simulink model "Test_9_bus_system"  (R2023b)
settings: Solver=VariableStepAuto  StartTime=0.0  StopTime=1  RelTol=1e-3
libraries: spsThreePhaseVIMeasurementLib x15, spsLoadFlowBusLib x9, spsPMUPLLBasedPositiveSequenceLib x6, spsSequenceAnalyzerLib x6, spsThreePhasePISectionLineLib x6, spsThreePhaseFaultLib x6, spsThreePhaseSourceLib x3, spsThreePhaseTransformerTwoWindingsLib x3, spsThreePhaseParallelRLCLoadLib x3, sps_lib x1
settings Model: Creator=korar  LastModifiedBy=korar

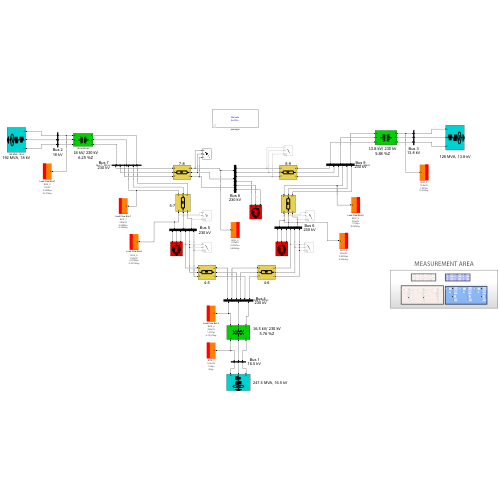
[thumbnail: Simulink's stored preview of the top-level diagram]
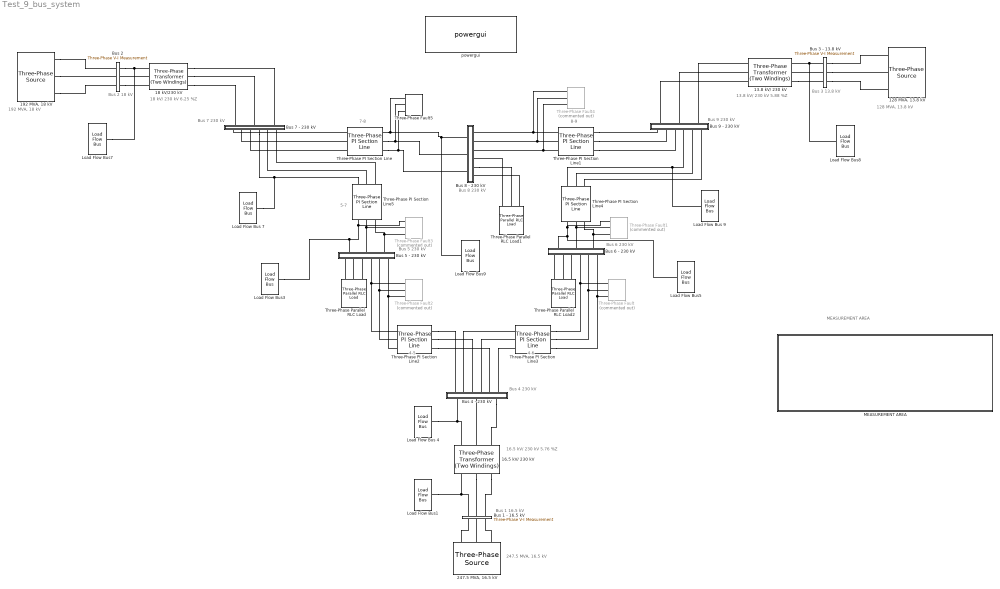
== system Test_9_bus_system ==
  note: MEASUREMENT AREA
  note: Bus 9
      | 230 kV
  note: 5-7
  note: 192 MVA, 18 kV
  note: 128 MVA, 13.8 kV
  note: 247.5 MVA, 16.5 kV
  note: 18 kV/ 230 kV
      | 6.25 %Z
  note: Bus 2
      | 18 kV
  note: Bus 3
      | 13.8 kV
  note: 13.8 kV/ 230 kV
      | 5.88 %Z
  note: Bus 1
      | 16.5 kV
  note: 16.5 kV/ 230 kV
      | 5.76 %Z
  note: 7-8
  note: 8-9
  note: 4-5
  note: 4-6
  note: Bus 7
      | 230 kV
  note: Bus 4
      | 230 kV
  note: Bus 5
      | 230 kV
  note: Bus 6
      | 230 kV
  note: Bus 8
      | 230 kV
  "128 MVA, 13.8 kV" : spsThreePhaseSourceLib/Three-Phase Source  InternalConnection=Yg  VoltagePhases=off  Voltage=(13800)*3.87688  PhaseAngle=72.604  Voltage_phases=[13.8e3 13.8e3 13.8e3]/sqrt(3)  PhaseAngles_phases=[0 -120 +120]  Frequency=50  NonIdealSource=on  SpecifyImpedance=off  Resistance=0.8929  Inductance=16.58e-3  ShortCircuitLevel=100e6  BaseVoltage=13.8e3  XRratio=7  BusType=PQ  Pref=128000000  Qref=11450000  Prefabc=[10e3, 10e3, 10e3]  Qrefabc=[0, 0, 0]  Qmin=-Inf  Qmax=Inf
  13.8 kV/ 230 kV : spsThreePhaseTransformerTwoWindingsLib/Three-Phase Transformer (Two Windings)  Winding1Connection=Yg  Winding2Connection=Yg  CoreType=Three single-phase transformers  SetSaturation=off  Hysteresis=off  DataFile='hysteresis'  SetInitialFlux=off  Measurements=None  UNITS=pu  NominalPower=[ 100e6 , 50 ]  Winding1=[ 13.8e3 , 1e-6 , 0 ]  Winding2=[ 230e3 , 1e-6 , 0.0586 ]  Rm=500  Lm=500  L0=0.5  Saturation=[ 0,0 ; 0.0024,1.2 ; 1.0,1.52 ]  InitialFluxes=[ 0.8 , -0.8 , 0.7 ]  BreakLoop=off  DiscreteSolver=Trapezoidal iterative  DataType=off  TransfoNumber=1
  16.5 kV/ 230 kV : spsThreePhaseTransformerTwoWindingsLib/Three-Phase Transformer (Two Windings)  Winding1Connection=Yg  Winding2Connection=Yg  CoreType=Three single-phase transformers  SetSaturation=off  Hysteresis=off  DataFile='hysteresis'  SetInitialFlux=off  Measurements=None  UNITS=pu  NominalPower=[ 100e6 , 50 ]  Winding1=[ 16.5e3 , 1e-6 , 0 ]  Winding2=[ 230e3 , 1e-6 , 0.0576 ]  Rm=500  Lm=500  L0=0.5  Saturation=[ 0,0 ; 0.0024,1.2 ; 1.0,1.52 ]  InitialFluxes=[ 0.8 , -0.8 , 0.7 ]  BreakLoop=off  DiscreteSolver=Trapezoidal iterative  DataType=off  TransfoNumber=1
  18 kV/230 kV : spsThreePhaseTransformerTwoWindingsLib/Three-Phase Transformer (Two Windings)  Winding1Connection=Yg  Winding2Connection=Yg  CoreType=Three single-phase transformers  SetSaturation=off  Hysteresis=off  DataFile='hysteresis'  SetInitialFlux=off  Measurements=None  UNITS=pu  NominalPower=[ 100e6 , 50 ]  Winding1=[ 18e3 , 1e-6 , 0 ]  Winding2=[ 230e3 , 1e-6 , 0.0625 ]  Rm=500  Lm=500  L0=0.5  Saturation=[ 0,0 ; 0.0024,1.2 ; 1.0,1.52 ]  InitialFluxes=[ 0.8 , -0.8 , 0.7 ]  BreakLoop=off  DiscreteSolver=Trapezoidal iterative  DataType=off  TransfoNumber=1
  "192 MVA, 18 kV" : spsThreePhaseSourceLib/Three-Phase Source  Description=|  InternalConnection=Yg  VoltagePhases=off  Voltage=(18000)*3.48427  PhaseAngle=78.8297  Voltage_phases=[13.8e3 13.8e3 13.8e3]/sqrt(3)  PhaseAngles_phases=[0 -120 +120]  Frequency=50  NonIdealSource=on  SpecifyImpedance=off  Resistance=0.8929  Inductance=16.58e-3  ShortCircuitLevel=100e6  BaseVoltage=18e3  XRratio=7  BusType=PQ  Pref=192000000  Qref=4900000  Prefabc=[10e3, 10e3, 10e3]  Qrefabc=[0, 0, 0]  Qmin=-Inf  Qmax=Inf
      | 60 MVA
      | 13.8 kV
  "247.5 MVA, 16.5 kV" : spsThreePhaseSourceLib/Three-Phase Source  Description=|  InternalConnection=Yg  VoltagePhases=off  Voltage=(16500)*2.16741  PhaseAngle=-2.7069  Voltage_phases=[13.8e3 13.8e3 13.8e3]/sqrt(3)  PhaseAngles_phases=[0 -120 +120]  Frequency=50  NonIdealSource=on  SpecifyImpedance=off  Resistance=0.8929  Inductance=16.58e-3  ShortCircuitLevel=100e6  BaseVoltage=16.5e3  XRratio=7  BusType=swing  Pref=247500000  Qref=27910000  Prefabc=[10e3, 10e3, 10e3]  Qrefabc=[0, 0, 0]  Qmin=-Inf  Qmax=Inf
      | 60 MVA
      | 13.8 kV
  Bus 1 - 16.5 kV : spsThreePhaseVIMeasurementLib/Three-Phase V-I Measurement  VoltageMeasurement=phase-to-ground  SetLabelV=on  LabelV=Vabc_1  Vpu=on  VpuLL=off  CurrentMeasurement=yes  SetLabelI=on  LabelI=Iabc_1  Ipu=on  Pbase=100e6  Vbase=16.5e3  OutputType=Complex  PhasorSimulation=off  PSBequivalent=0
  Bus 2 : spsThreePhaseVIMeasurementLib/Three-Phase V-I Measurement  VoltageMeasurement=phase-to-ground  SetLabelV=on  LabelV=Vabc_2  Vpu=on  VpuLL=off  CurrentMeasurement=yes  SetLabelI=on  LabelI=Iabc_2  Ipu=on  Pbase=100e6  Vbase=18e3  OutputType=Complex  PhasorSimulation=off  PSBequivalent=0
  Bus 3 - 13.8 kV : spsThreePhaseVIMeasurementLib/Three-Phase V-I Measurement  VoltageMeasurement=phase-to-ground  SetLabelV=on  LabelV=Vabc_3  Vpu=on  VpuLL=off  CurrentMeasurement=yes  SetLabelI=on  LabelI=Iabc_3  Ipu=on  Pbase=100e6  Vbase=13.8e3  OutputType=Complex  PhasorSimulation=off  PSBequivalent=0
  Bus 4 - 230 kV : Subsystem
  Bus 5 - 230 kV : Subsystem
  Bus 6 - 230 kV : Subsystem
  Bus 7 - 230 kV : Subsystem
  Bus 8 - 230 kV : Subsystem
  Bus 9 - 230 kV : Subsystem
  Load Flow Bus 4 : spsLoadFlowBusLib/Load Flow Bus  LConnTagsString=a  Phases=single  Connectors=on one side  ID=BUS_4  Vbase=230e3  Vref=1  Vangle=0  VLF=1.007  VLFb=1  VLFc=1  angleLF=-0.1437  angleLFb=0  angleLFc=0
  Load Flow Bus 7 : spsLoadFlowBusLib/Load Flow Bus  LConnTagsString=a  Phases=single  Connectors=on one side  ID=BUS_7  Vbase=230e3  Vref=1  Vangle=0  VLF=0.9982  VLFb=1  VLFc=1  angleLF=9.326  angleLFb=0  angleLFc=0
  Load Flow Bus 9 : spsLoadFlowBusLib/Load Flow Bus  LConnTagsString=a  Phases=single  Connectors=on one side  ID=BUS_9  Vbase=230e3  Vref=1  Vangle=0  VLF=1.019  VLFb=1  VLFc=1  angleLF=8.097  angleLFb=0  angleLFc=0
  Load Flow Bus1 : spsLoadFlowBusLib/Load Flow Bus  LConnTagsString=a  Phases=single  Connectors=on one side  ID=BUS_1  Vbase=16.5e3  Vref=1.04  Vangle=0  VLF=1.04  VLFb=1  VLFc=1  angleLF=0  angleLFb=0  angleLFc=0
  Load Flow Bus3 : spsLoadFlowBusLib/Load Flow Bus  LConnTagsString=a  Phases=single  Connectors=on one side  ID=BUS_5  Vbase=230e3  Vref=1  Vangle=0  VLF=0.9705  VLFb=1  VLFc=1  angleLF=-0.2218  angleLFb=0  angleLFc=0
  Load Flow Bus5 : spsLoadFlowBusLib/Load Flow Bus  LConnTagsString=a  Phases=single  Connectors=on one side  ID=BUS_6  Vbase=230e3  Vref=1  Vangle=0  VLF=0.9908  VLFb=1  VLFc=1  angleLF=0.264  angleLFb=0  angleLFc=0
  Load Flow Bus7 : spsLoadFlowBusLib/Load Flow Bus  LConnTagsString=a  Phases=single  Connectors=on one side  ID=BUS_2  Vbase=18e3  Vref=1.025  Vangle=0  VLF=0.9938  VLFb=1  VLFc=1  angleLF=16.27  angleLFb=0  angleLFc=0
  Load Flow Bus8 : spsLoadFlowBusLib/Load Flow Bus  LConnTagsString=a  Phases=single  Connectors=on one side  ID=BUS_3  Vbase=13.8e3  Vref=1.025  Vangle=0  VLF=1.023  VLFb=1  VLFc=1  angleLF=12.22  angleLFb=0  angleLFc=0
  Load Flow Bus9 : spsLoadFlowBusLib/Load Flow Bus  LConnTagsString=a  Phases=single  Connectors=on one side  ID=BUS_8  Vbase=230e3  Vref=1  Vangle=0  VLF=0.9941  VLFb=1  VLFc=1  angleLF=6.865  angleLFb=0  angleLFc=0
  MEASUREMENT AREA : Subsystem
  Three-Phase PI Section Line : spsThreePhasePISectionLineLib/Three-Phase PI Section Line  LConnTagsString=a|b|c  RConnTagsString=A|B|C  Length=100  Frequency=50  Resistances=[ 0.044965 0.11241]  Inductances="[ 1.01e-3  2.02e-3]"  Capacitances=[7.471e-9 4.394e-9]
  Three-Phase PI Section Line1 : spsThreePhasePISectionLineLib/Three-Phase PI Section Line  LConnTagsString=a|b|c  RConnTagsString=A|B|C  Length=100  Frequency=50  Resistances=[ 0.062951 0.15737]  Inductances="[ 1.414e-3  3.53e-3]"  Capacitances=[10.47e-9 6.15e-9]
  Three-Phase PI Section Line2 : spsThreePhasePISectionLineLib/Three-Phase PI Section Line  LConnTagsString=a|b|c  RConnTagsString=A|B|C  Length=100  Frequency=50  Resistances=[ 0.0529 0.13225]  Inductances="[ 1.192e-3  2.38e-3]"  Capacitances=[8.82e-9 5.188e-9]
  Three-Phase PI Section Line3 : spsThreePhasePISectionLineLib/Three-Phase PI Section Line  LConnTagsString=a|b|c  RConnTagsString=A|B|C  Length=100  Frequency=50  Resistances=[ 0.08993 0.224825]  Inductances="[ 1.29e-3  3.22e-3]"  Capacitances=[7.922e-9 4.74e-9]
  Three-Phase PI Section Line4 : spsThreePhasePISectionLineLib/Three-Phase PI Section Line  LConnTagsString=a|b|c  RConnTagsString=A|B|C  Length=100  Frequency=50  Resistances=[ 0.20631 0.5157]  Inductances="[ 2.38e-3  6.09e-3]"  Capacitances=[17.95e-9 10.55e-9]
  Three-Phase PI Section Line5 : spsThreePhasePISectionLineLib/Three-Phase PI Section Line  LConnTagsString=a|b|c  RConnTagsString=A|B|C  Length=100  Frequency=50  Resistances=[ 0.16928 0.4232]  Inductances="[ 2.259e-3  5.64e-3]"  Capacitances=[15.34e-9 9.025e-9]
  Three-Phase Parallel RLC Load : spsThreePhaseParallelRLCLoadLib/Three-Phase Parallel RLC Load  LConnTagsString=A|B|C  Configuration=Y (grounded)  NominalVoltage=(230000)*0.970466  Vabc=[1e3 1e3 1e3]  Vabcp=[1e3 1e3 1e3]  NominalFrequency=50  UnbalancedPower=off  ActivePower=125000000  InductivePower=50000000  CapacitivePower=0  Pabc=[10e3 9e3 11e3]  QLabc=[100 90 110]  QCabc=[100 90 110]  Pabcp=[10e3 9e3 11e3]  QLabcp=[100 90 110]  QCabcp=[100 90 110]  Measurements=None  LoadType=constant PQ
  Three-Phase Parallel RLC Load1 : spsThreePhaseParallelRLCLoadLib/Three-Phase Parallel RLC Load  LConnTagsString=A|B|C  Configuration=Y (grounded)  NominalVoltage=(230000)*0.994116  Vabc=[1e3 1e3 1e3]  Vabcp=[1e3 1e3 1e3]  NominalFrequency=50  UnbalancedPower=off  ActivePower=100000000  InductivePower=35000000  CapacitivePower=0  Pabc=[10e3 9e3 11e3]  QLabc=[100 90 110]  QCabc=[100 90 110]  Pabcp=[10e3 9e3 11e3]  QLabcp=[100 90 110]  QCabcp=[100 90 110]  Measurements=None  LoadType=constant PQ
  Three-Phase Parallel RLC Load2 : spsThreePhaseParallelRLCLoadLib/Three-Phase Parallel RLC Load  LConnTagsString=A|B|C  Configuration=Y (grounded)  NominalVoltage=(230000)*0.990813  Vabc=[1e3 1e3 1e3]  Vabcp=[1e3 1e3 1e3]  NominalFrequency=50  UnbalancedPower=off  ActivePower=90000000  InductivePower=30000000  CapacitivePower=0  Pabc=[10e3 9e3 11e3]  QLabc=[100 90 110]  QCabc=[100 90 110]  Pabcp=[10e3 9e3 11e3]  QLabcp=[100 90 110]  QCabcp=[100 90 110]  Measurements=None  LoadType=constant PQ
  Three-Phase Fault : spsThreePhaseFaultLib/Three-Phase Fault  Commented=on  InitialStates=0  FaultA=on  FaultB=on  FaultC=on  GroundFault=on  SwitchTimes="[0.6  1]"  External=off  SwitchStatus=NaN  FaultResistance=0.001  GroundResistance=0.01  SnubberResistance=1e6  SnubberCapacitance=inf  Measurements=Fault currents
  Three-Phase Fault1 : spsThreePhaseFaultLib/Three-Phase Fault  Commented=on  InitialStates=0  FaultA=on  FaultB=off  FaultC=off  GroundFault=on  SwitchTimes="[0.6  1]"  External=off  SwitchStatus=NaN  FaultResistance=0.001  GroundResistance=0.01  SnubberResistance=1e6  SnubberCapacitance=inf  Measurements=Fault currents
  Three-Phase Fault2 : spsThreePhaseFaultLib/Three-Phase Fault  Commented=on  InitialStates=0  FaultA=off  FaultB=on  FaultC=on  GroundFault=off  SwitchTimes="[8  10]"  External=off  SwitchStatus=NaN  FaultResistance=0.001  GroundResistance=0.01  SnubberResistance=1e6  SnubberCapacitance=inf  Measurements=Fault currents
  Three-Phase Fault3 : spsThreePhaseFaultLib/Three-Phase Fault  Commented=on  InitialStates=0  FaultA=off  FaultB=on  FaultC=on  GroundFault=off  SwitchTimes="[6/10  1]"  External=off  SwitchStatus=NaN  FaultResistance=0.001  GroundResistance=0.01  SnubberResistance=1e6  SnubberCapacitance=inf  Measurements=Fault currents
  Three-Phase Fault4 : spsThreePhaseFaultLib/Three-Phase Fault  Commented=on  InitialStates=0  FaultA=on  FaultB=on  FaultC=on  GroundFault=off  SwitchTimes="[8  10]"  External=off  SwitchStatus=NaN  FaultResistance=0.001  GroundResistance=0.01  SnubberResistance=1e6  SnubberCapacitance=inf  Measurements=Fault currents
  Three-Phase Fault5 : spsThreePhaseFaultLib/Three-Phase Fault  InitialStates=0  FaultA=off  FaultB=on  FaultC=on  GroundFault=off  SwitchTimes="[0.6  1]"  External=off  SwitchStatus=NaN  FaultResistance=0.001  GroundResistance=0.01  SnubberResistance=1e6  SnubberCapacitance=inf  Measurements=Fault currents
  powergui : sps_lib/powergui  Priority=1  SimulationMode=Discrete  SampleTime=50e-6  frequency=50  Iterations=50  frequencyindice=50  Pbase=100e6  ErrMax=1e-4  UnitsV=kV  UnitsW=MW  buscounter=0  FunctionMessages=off  echomessages=off  EnableUseOfTLC=off  CurrentSourceSwitches=off  DisableSnubberDevices=off  DisableRonSwitches=off  DisableVfSwitches=off  DisplayEquations=off  AutomaticDiscreteSolvers=off  SolverType=Tustin/Backward Euler (TBE)  Interpol=off  ExternalGateDelay=off  methode=off  Ts=100  x0status=blocks  SPID=on  SwTol=0  HookPort=off  NonlinearTolerance=1e-4  nMaxIteration=100  ContinueOnMaxIteration=off  RestoreLinks=warning  ResistiveCurrentMeasurement=off  Frange=[0:2:500]  Ylog=off  Xlog=on  ShowGrid=off  save=off  variable=ZData  structure=0  ZoomFFT=off  StartTime=0.0  cycles=1  DisplayStyle=1  fundamental=60  FreqAxis=off  MaxFrequency=1000  frequencyindicesteady=1  RmsSteady=1  display=off
  connections:
  Bus 3 - 13.8 kV/RConn1 -- "128 MVA, 13.8 kV"/RConn1
  Bus 3 - 13.8 kV/RConn2 -- "128 MVA, 13.8 kV"/RConn2
  Bus 3 - 13.8 kV/RConn3 -- "128 MVA, 13.8 kV"/RConn3
  "247.5 MVA, 16.5 kV"/RConn1 -- Bus 1 - 16.5 kV/RConn1
  "247.5 MVA, 16.5 kV"/RConn2 -- Bus 1 - 16.5 kV/RConn2
  "247.5 MVA, 16.5 kV"/RConn3 -- Bus 1 - 16.5 kV/RConn3
  Three-Phase PI Section Line/LConn1 -- Bus 7 - 230 kV/RConn1
  Three-Phase PI Section Line/LConn2 -- Bus 7 - 230 kV/RConn2
  Three-Phase PI Section Line/LConn3 -- Bus 7 - 230 kV/RConn3
  Bus 7 - 230 kV/RConn4 -- Load Flow Bus 7/LConn1 -- Three-Phase PI Section Line5/LConn1
  Three-Phase PI Section Line5/LConn2 -- Bus 7 - 230 kV/RConn5
  Three-Phase PI Section Line5/LConn3 -- Bus 7 - 230 kV/RConn6
  "192 MVA, 18 kV"/RConn1 -- Bus 2/LConn1
  "192 MVA, 18 kV"/RConn2 -- Bus 2/LConn2
  "192 MVA, 18 kV"/RConn3 -- Bus 2/LConn3
  Three-Phase PI Section Line1/RConn1 -- Bus 9 - 230 kV/LConn1
  Three-Phase PI Section Line1/RConn2 -- Bus 9 - 230 kV/LConn2
  Three-Phase PI Section Line1/RConn3 -- Bus 9 - 230 kV/LConn3
  Three-Phase PI Section Line4/LConn1 -- Load Flow Bus 9/LConn1 -- Bus 9 - 230 kV/LConn4
  Three-Phase PI Section Line4/LConn2 -- Bus 9 - 230 kV/LConn5
  Three-Phase PI Section Line4/LConn3 -- Bus 9 - 230 kV/LConn6
  Three-Phase PI Section Line2/RConn1 -- Bus 4 - 230 kV/RConn1
  Three-Phase PI Section Line3/LConn1 -- Bus 4 - 230 kV/RConn2
  Three-Phase PI Section Line2/RConn2 -- Bus 4 - 230 kV/RConn3
  Three-Phase PI Section Line3/LConn2 -- Bus 4 - 230 kV/RConn4
  Three-Phase PI Section Line2/RConn3 -- Bus 4 - 230 kV/RConn5
  Three-Phase PI Section Line3/LConn3 -- Bus 4 - 230 kV/RConn6
  Three-Phase PI Section Line5/RConn2 -- Bus 5 - 230 kV/LConn2 -- Three-Phase Fault3/LConn2
  Three-Phase PI Section Line2/LConn1 -- Three-Phase Fault2/LConn1 -- Bus 5 - 230 kV/RConn4
  Three-Phase PI Section Line2/LConn2 -- Three-Phase Fault2/LConn2 -- Bus 5 - 230 kV/RConn5
  Three-Phase PI Section Line2/LConn3 -- Three-Phase Fault2/LConn3 -- Bus 5 - 230 kV/RConn6
  Three-Phase PI Section Line4/RConn1 -- Load Flow Bus5/LConn1 -- Bus 6 - 230 kV/LConn1 -- Three-Phase Fault1/LConn1
  Three-Phase PI Section Line4/RConn2 -- Bus 6 - 230 kV/LConn2 -- Three-Phase Fault1/LConn2
  Three-Phase PI Section Line4/RConn3 -- Bus 6 - 230 kV/LConn3 -- Three-Phase Fault1/LConn3
  Three-Phase PI Section Line3/RConn1 -- Three-Phase Fault/LConn1 -- Bus 6 - 230 kV/RConn4
  Three-Phase PI Section Line3/RConn2 -- Three-Phase Fault/LConn2 -- Bus 6 - 230 kV/RConn5
  Three-Phase PI Section Line3/RConn3 -- Three-Phase Fault/LConn3 -- Bus 6 - 230 kV/RConn6
  18 kV/230 kV/RConn2 -- Bus 7 - 230 kV/LConn2
  18 kV/230 kV/RConn1 -- Bus 7 - 230 kV/LConn3
  18 kV/230 kV/RConn3 -- Bus 7 - 230 kV/LConn1
  Bus 2/RConn1 -- Load Flow Bus7/LConn1 -- 18 kV/230 kV/LConn1
  Bus 2/RConn3 -- 18 kV/230 kV/LConn3
  18 kV/230 kV/LConn2 -- Bus 2/RConn2
  Bus 9 - 230 kV/RConn1 -- 13.8 kV/ 230 kV/RConn3
  Bus 3 - 13.8 kV/LConn1 -- Load Flow Bus8/LConn1 -- 13.8 kV/ 230 kV/LConn1
  Bus 3 - 13.8 kV/LConn2 -- 13.8 kV/ 230 kV/LConn2
  13.8 kV/ 230 kV/LConn3 -- Bus 3 - 13.8 kV/LConn3
  13.8 kV/ 230 kV/RConn1 -- Bus 9 - 230 kV/RConn3
  13.8 kV/ 230 kV/RConn2 -- Bus 9 - 230 kV/RConn2
  16.5 kV/ 230 kV/RConn2 -- Bus 4 - 230 kV/LConn2
  16.5 kV/ 230 kV/RConn1 -- Load Flow Bus 4/LConn1 -- Bus 4 - 230 kV/LConn1
  Bus 4 - 230 kV/LConn3 -- 16.5 kV/ 230 kV/RConn3
  16.5 kV/ 230 kV/LConn2 -- Bus 1 - 16.5 kV/LConn2
  16.5 kV/ 230 kV/LConn3 -- Bus 1 - 16.5 kV/LConn3
  Bus 1 - 16.5 kV/LConn1 -- Load Flow Bus1/LConn1 -- 16.5 kV/ 230 kV/LConn1
  Three-Phase PI Section Line/RConn1 -- Three-Phase Fault5/LConn1 -- Load Flow Bus9/LConn1 -- Bus 8 - 230 kV/LConn1
  Three-Phase PI Section Line1/LConn1 -- Three-Phase Fault4/LConn1 -- Bus 8 - 230 kV/RConn1
  Three-Phase PI Section Line/RConn2 -- Three-Phase Fault5/LConn2 -- Bus 8 - 230 kV/LConn2
  Three-Phase PI Section Line1/LConn2 -- Three-Phase Fault4/LConn2 -- Bus 8 - 230 kV/RConn2
  Three-Phase PI Section Line/RConn3 -- Three-Phase Fault5/LConn3 -- Bus 8 - 230 kV/LConn3
  Three-Phase PI Section Line1/LConn3 -- Three-Phase Fault4/LConn3 -- Bus 8 - 230 kV/RConn3
  Bus 5 - 230 kV/LConn1 -- Load Flow Bus3/LConn1 -- Three-Phase Fault3/LConn1 -- Three-Phase PI Section Line5/RConn1
  Bus 5 - 230 kV/LConn3 -- Three-Phase PI Section Line5/RConn3 -- Three-Phase Fault3/LConn3
  Three-Phase Parallel RLC Load/LConn1 -- Bus 5 - 230 kV/RConn1
  Three-Phase Parallel RLC Load/LConn2 -- Bus 5 - 230 kV/RConn2
  Three-Phase Parallel RLC Load/LConn3 -- Bus 5 - 230 kV/RConn3
  Three-Phase Parallel RLC Load1/LConn1 -- Bus 8 - 230 kV/RConn4
  Bus 8 - 230 kV/RConn5 -- Three-Phase Parallel RLC Load1/LConn2
  Three-Phase Parallel RLC Load1/LConn3 -- Bus 8 - 230 kV/RConn6
  Three-Phase Parallel RLC Load2/LConn1 -- Bus 6 - 230 kV/RConn1
  Three-Phase Parallel RLC Load2/LConn2 -- Bus 6 - 230 kV/RConn2
  Three-Phase Parallel RLC Load2/LConn3 -- Bus 6 - 230 kV/RConn3

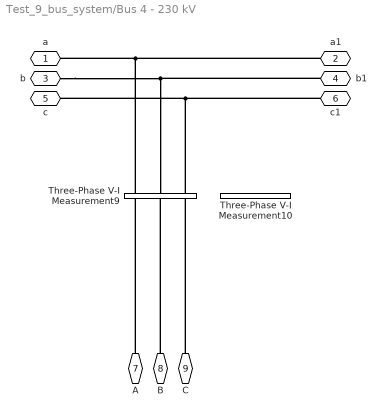
== system Test_9_bus_system/Bus 4 - 230 kV ==
  Three-Phase V-I Measurement10 : spsThreePhaseVIMeasurementLib/Three-Phase V-I Measurement  VoltageMeasurement=phase-to-ground  SetLabelV=on  LabelV=Vabc_42  Vpu=on  VpuLL=off  CurrentMeasurement=yes  SetLabelI=on  LabelI=Iabc_42  Ipu=on  Pbase=100e6  Vbase=230e3  OutputType=Complex  PhasorSimulation=off  PSBequivalent=0
  Three-Phase V-I Measurement9 : spsThreePhaseVIMeasurementLib/Three-Phase V-I Measurement  VoltageMeasurement=phase-to-ground  SetLabelV=on  LabelV=Vabc_41  Vpu=on  VpuLL=off  CurrentMeasurement=yes  SetLabelI=on  LabelI=Iabc_41  Ipu=on  Pbase=100e6  Vbase=230e3  OutputType=Complex  PhasorSimulation=off  PSBequivalent=0
  a : PMIOPort  Side=Right
  a1 : PMIOPort  Port=2  Side=Right
  b : PMIOPort  Port=3  Side=Right
  b1 : PMIOPort  Port=4  Side=Right
  c : PMIOPort  Port=5  Side=Right
  c1 : PMIOPort  Port=6  Side=Right
  A : PMIOPort  Port=7  Side=Left
  B : PMIOPort  Port=8  Side=Left
  C : PMIOPort  Port=9  Side=Left
  connections:
  B/RConn1 -- Three-Phase V-I Measurement9/LConn2
  C/RConn1 -- Three-Phase V-I Measurement9/LConn3
  Three-Phase V-I Measurement9/RConn3 -- c1/RConn1 -- c/RConn1
  A/RConn1 -- Three-Phase V-I Measurement9/LConn1
  b/RConn1 -- b1/RConn1 -- Three-Phase V-I Measurement9/RConn2
  Three-Phase V-I Measurement9/RConn1 -- a1/RConn1 -- a/RConn1

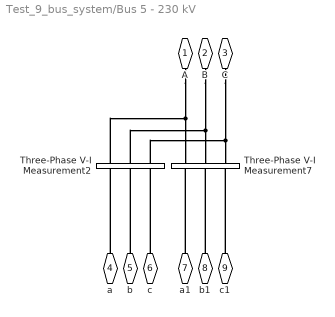
== system Test_9_bus_system/Bus 5 - 230 kV ==
  Three-Phase V-I Measurement2 : spsThreePhaseVIMeasurementLib/Three-Phase V-I Measurement  VoltageMeasurement=phase-to-ground  SetLabelV=on  LabelV=Vabc_51  Vpu=on  VpuLL=off  CurrentMeasurement=yes  SetLabelI=on  LabelI=Iabc_51  Ipu=on  Pbase=100e6  Vbase=230e3  OutputType=Complex  PhasorSimulation=off  PSBequivalent=0
  Three-Phase V-I Measurement7 : spsThreePhaseVIMeasurementLib/Three-Phase V-I Measurement  VoltageMeasurement=phase-to-ground  SetLabelV=on  LabelV=Vabc_52  Vpu=on  VpuLL=off  CurrentMeasurement=yes  SetLabelI=on  LabelI=Iabc_52  Ipu=on  Pbase=100e6  Vbase=230e3  OutputType=Complex  PhasorSimulation=off  PSBequivalent=0
  A : PMIOPort  Side=Left
  B : PMIOPort  Port=2  Side=Left
  C : PMIOPort  Port=3  Side=Left
  a : PMIOPort  Port=4  Side=Right
  b : PMIOPort  Port=5  Side=Right
  c : PMIOPort  Port=6  Side=Right
  a1 : PMIOPort  Port=7  Side=Right
  b1 : PMIOPort  Port=8  Side=Right
  c1 : PMIOPort  Port=9  Side=Right
  connections:
  B/RConn1 -- Three-Phase V-I Measurement2/LConn2 -- Three-Phase V-I Measurement7/LConn2
  b/RConn1 -- Three-Phase V-I Measurement2/RConn2
  A/RConn1 -- Three-Phase V-I Measurement2/LConn1 -- Three-Phase V-I Measurement7/LConn1
  a/RConn1 -- Three-Phase V-I Measurement2/RConn1
  a1/RConn1 -- Three-Phase V-I Measurement7/RConn1
  c1/RConn1 -- Three-Phase V-I Measurement7/RConn3
  C/RConn1 -- Three-Phase V-I Measurement2/LConn3 -- Three-Phase V-I Measurement7/LConn3
  b1/RConn1 -- Three-Phase V-I Measurement7/RConn2
  c/RConn1 -- Three-Phase V-I Measurement2/RConn3

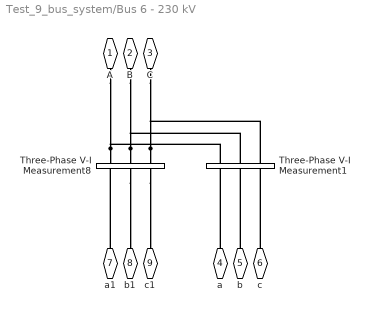
== system Test_9_bus_system/Bus 6 - 230 kV ==
  Three-Phase V-I Measurement1 : spsThreePhaseVIMeasurementLib/Three-Phase V-I Measurement  VoltageMeasurement=phase-to-ground  SetLabelV=on  LabelV=Vabc_62  Vpu=on  VpuLL=off  CurrentMeasurement=yes  SetLabelI=on  LabelI=Iabc_62  Ipu=on  Pbase=100e6  Vbase=230e3  OutputType=Complex  PhasorSimulation=off  PSBequivalent=0
  Three-Phase V-I Measurement8 : spsThreePhaseVIMeasurementLib/Three-Phase V-I Measurement  VoltageMeasurement=phase-to-ground  SetLabelV=on  LabelV=Vabc_61  Vpu=on  VpuLL=off  CurrentMeasurement=yes  SetLabelI=on  LabelI=Iabc_61  Ipu=on  Pbase=100e6  Vbase=230e3  OutputType=Complex  PhasorSimulation=off  PSBequivalent=0
  A : PMIOPort  Side=Left
  B : PMIOPort  Port=2  Side=Left
  C : PMIOPort  Port=3  Side=Left
  a : PMIOPort  Port=4  Side=Right
  b : PMIOPort  Port=5  Side=Right
  c : PMIOPort  Port=6  Side=Right
  a1 : PMIOPort  Port=7  Side=Right
  b1 : PMIOPort  Port=8  Side=Right
  c1 : PMIOPort  Port=9  Side=Right
  connections:
  Three-Phase V-I Measurement8/LConn2 -- B/RConn1 -- Three-Phase V-I Measurement1/LConn2
  Three-Phase V-I Measurement8/LConn1 -- A/RConn1 -- Three-Phase V-I Measurement1/LConn1
  b/RConn1 -- Three-Phase V-I Measurement1/RConn2
  Three-Phase V-I Measurement8/LConn3 -- C/RConn1 -- Three-Phase V-I Measurement1/LConn3
  a/RConn1 -- Three-Phase V-I Measurement1/RConn1
  Three-Phase V-I Measurement8/RConn3 -- c1/RConn1
  Three-Phase V-I Measurement8/RConn2 -- b1/RConn1
  c/RConn1 -- Three-Phase V-I Measurement1/RConn3
  a1/RConn1 -- Three-Phase V-I Measurement8/RConn1

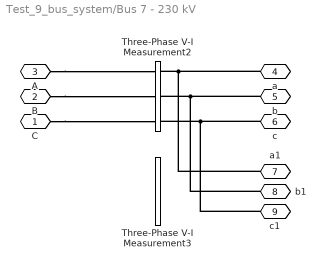
== system Test_9_bus_system/Bus 7 - 230 kV ==
  Three-Phase V-I Measurement2 : spsThreePhaseVIMeasurementLib/Three-Phase V-I Measurement  VoltageMeasurement=phase-to-ground  SetLabelV=on  LabelV=Vabc_71  Vpu=on  VpuLL=off  CurrentMeasurement=yes  SetLabelI=on  LabelI=Iabc_71  Ipu=on  Pbase=100e6  Vbase=230e3  OutputType=Complex  PhasorSimulation=off  PSBequivalent=0
  Three-Phase V-I Measurement3 : spsThreePhaseVIMeasurementLib/Three-Phase V-I Measurement  VoltageMeasurement=phase-to-ground  SetLabelV=on  LabelV=Vabc_72  Vpu=on  VpuLL=off  CurrentMeasurement=yes  SetLabelI=on  LabelI=Iabc_72  Ipu=on  Pbase=100e6  Vbase=230e3  OutputType=Complex  PhasorSimulation=off  PSBequivalent=0
  C : PMIOPort  Side=Left
  B : PMIOPort  Port=2  Side=Left
  A : PMIOPort  Port=3  Side=Left
  a : PMIOPort  Port=4  Side=Right
  b : PMIOPort  Port=5  Side=Right
  c : PMIOPort  Port=6  Side=Right
  a1 : PMIOPort  Port=7  Side=Right
  b1 : PMIOPort  Port=8  Side=Right
  c1 : PMIOPort  Port=9  Side=Right
  connections:
  C/RConn1 -- Three-Phase V-I Measurement2/LConn3
  a/RConn1 -- a1/RConn1 -- Three-Phase V-I Measurement2/RConn1
  A/RConn1 -- Three-Phase V-I Measurement2/LConn1
  b/RConn1 -- b1/RConn1 -- Three-Phase V-I Measurement2/RConn2
  B/RConn1 -- Three-Phase V-I Measurement2/LConn2
  c/RConn1 -- c1/RConn1 -- Three-Phase V-I Measurement2/RConn3

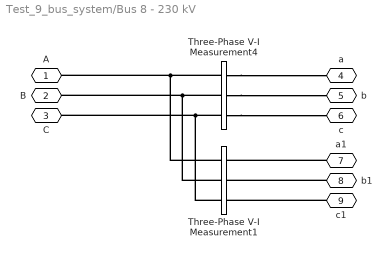
== system Test_9_bus_system/Bus 8 - 230 kV ==
  Three-Phase V-I Measurement1 : spsThreePhaseVIMeasurementLib/Three-Phase V-I Measurement  VoltageMeasurement=phase-to-ground  SetLabelV=on  LabelV=Vabc_82  Vpu=on  VpuLL=off  CurrentMeasurement=yes  SetLabelI=on  LabelI=Iabc_82  Ipu=on  Pbase=100e6  Vbase=230e3  OutputType=Complex  PhasorSimulation=off  PSBequivalent=0
  Three-Phase V-I Measurement4 : spsThreePhaseVIMeasurementLib/Three-Phase V-I Measurement  VoltageMeasurement=phase-to-ground  SetLabelV=on  LabelV=Vabc_81  Vpu=on  VpuLL=off  CurrentMeasurement=yes  SetLabelI=on  LabelI=Iabc_81  Ipu=on  Pbase=100e6  Vbase=230e3  OutputType=Complex  PhasorSimulation=off  PSBequivalent=0
  A : PMIOPort  Side=Left
  B : PMIOPort  Port=2  Side=Left
  C : PMIOPort  Port=3  Side=Left
  a : PMIOPort  Port=4  Side=Right
  b : PMIOPort  Port=5  Side=Right
  c : PMIOPort  Port=6  Side=Right
  a1 : PMIOPort  Port=7  Side=Right
  b1 : PMIOPort  Port=8  Side=Right
  c1 : PMIOPort  Port=9  Side=Right
  connections:
  Three-Phase V-I Measurement4/LConn1 -- A/RConn1 -- Three-Phase V-I Measurement1/LConn1
  Three-Phase V-I Measurement4/RConn1 -- a/RConn1
  Three-Phase V-I Measurement4/LConn3 -- C/RConn1 -- Three-Phase V-I Measurement1/LConn3
  Three-Phase V-I Measurement4/LConn2 -- B/RConn1 -- Three-Phase V-I Measurement1/LConn2
  Three-Phase V-I Measurement4/RConn3 -- c/RConn1
  Three-Phase V-I Measurement4/RConn2 -- b/RConn1
  a1/RConn1 -- Three-Phase V-I Measurement1/RConn1
  b1/RConn1 -- Three-Phase V-I Measurement1/RConn2
  c1/RConn1 -- Three-Phase V-I Measurement1/RConn3

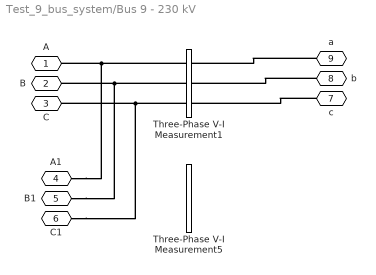
== system Test_9_bus_system/Bus 9 - 230 kV ==
  Three-Phase V-I Measurement1 : spsThreePhaseVIMeasurementLib/Three-Phase V-I Measurement  VoltageMeasurement=phase-to-ground  SetLabelV=on  LabelV=Vabc_91  Vpu=on  VpuLL=off  CurrentMeasurement=yes  SetLabelI=on  LabelI=Iabc_91  Ipu=on  Pbase=100e6  Vbase=230e3  OutputType=Complex  PhasorSimulation=off  PSBequivalent=0
  Three-Phase V-I Measurement5 : spsThreePhaseVIMeasurementLib/Three-Phase V-I Measurement  VoltageMeasurement=phase-to-ground  SetLabelV=on  LabelV=Vabc_92  Vpu=on  VpuLL=off  CurrentMeasurement=yes  SetLabelI=on  LabelI=Iabc_92  Ipu=on  Pbase=100e6  Vbase=230e3  OutputType=Complex  PhasorSimulation=off  PSBequivalent=0
  A : PMIOPort  Side=Left
  B : PMIOPort  Port=2  Side=Left
  C : PMIOPort  Port=3  Side=Left
  A1 : PMIOPort  Port=4  Side=Left
  B1 : PMIOPort  Port=5  Side=Left
  C1 : PMIOPort  Port=6  Side=Left
  c : PMIOPort  Port=7  Side=Right
  b : PMIOPort  Port=8  Side=Right
  a : PMIOPort  Port=9  Side=Right
  connections:
  Three-Phase V-I Measurement1/LConn1 -- A1/RConn1 -- A/RConn1
  b/RConn1 -- Three-Phase V-I Measurement1/RConn2
  Three-Phase V-I Measurement1/LConn3 -- C1/RConn1 -- C/RConn1
  c/RConn1 -- Three-Phase V-I Measurement1/RConn3
  a/RConn1 -- Three-Phase V-I Measurement1/RConn1
  Three-Phase V-I Measurement1/LConn2 -- B1/RConn1 -- B/RConn1

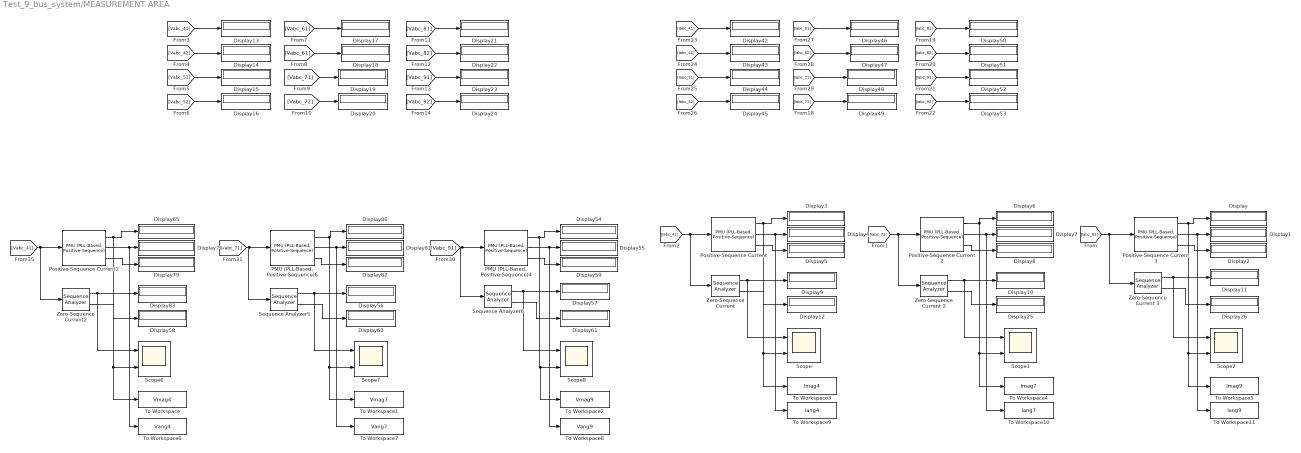
== system Test_9_bus_system/MEASUREMENT AREA ==
  Display{,1..26,42..61,65,76,79..83} (54 alike) : Display
  "PMU (PLL-Based, Positive-Sequence)4" : spsPMUPLLBasedPositiveSequenceLib/PMU (PLL-Based, Positive-Sequence)  nominalFrequency=50  samplingRate=64  reportingFactor=1
      settings: LibrarySourceBlock=|
      | sps_lib/Sensors and Measurements/PMU
      | (PLL-Based,
      | Positive-Sequence)
  "PMU (PLL-Based, Positive-Sequence)6" : spsPMUPLLBasedPositiveSequenceLib/PMU (PLL-Based, Positive-Sequence)  nominalFrequency=50  samplingRate=64  reportingFactor=1
      settings: LibrarySourceBlock=|
      | sps_lib/Sensors and Measurements/PMU
      | (PLL-Based,
      | Positive-Sequence)
  Positive-Sequence Current : spsPMUPLLBasedPositiveSequenceLib/PMU (PLL-Based, Positive-Sequence)  nominalFrequency=50  samplingRate=64  reportingFactor=1
      settings: LibrarySourceBlock=|
      | sps_lib/Sensors and Measurements/PMU
      | (PLL-Based,
      | Positive-Sequence)
  Positive-Sequence Current 2 : spsPMUPLLBasedPositiveSequenceLib/PMU (PLL-Based, Positive-Sequence)  nominalFrequency=50  samplingRate=64  reportingFactor=1
      settings: LibrarySourceBlock=|
      | sps_lib/Sensors and Measurements/PMU
      | (PLL-Based,
      | Positive-Sequence)
  Positive-Sequence Current 3 : spsPMUPLLBasedPositiveSequenceLib/PMU (PLL-Based, Positive-Sequence)  nominalFrequency=50  samplingRate=64  reportingFactor=1
      settings: LibrarySourceBlock=|
      | sps_lib/Sensors and Measurements/PMU
      | (PLL-Based,
      | Positive-Sequence)
  Positive-Sequence Current2 : spsPMUPLLBasedPositiveSequenceLib/PMU (PLL-Based, Positive-Sequence)  nominalFrequency=50  samplingRate=64  reportingFactor=1
      settings: LibrarySourceBlock=|
      | sps_lib/Sensors and Measurements/PMU
      | (PLL-Based,
      | Positive-Sequence)
  Scope{,1..2,6..8} (6 alike) : Scope  NumInputPorts=2
  Sequence Analyzer5 : spsSequenceAnalyzerLib/Sequence Analyzer  Freq=50  n=1  seq=Zero  InInit=[1, 0]  Ts=0
      settings: LibrarySourceBlock=sps_lib/Sensors and Measurements/Sequence Analyzer
  Sequence Analyzer6 : spsSequenceAnalyzerLib/Sequence Analyzer  Freq=50  n=1  seq=Zero  InInit=[1, 0]  Ts=0
      settings: LibrarySourceBlock=sps_lib/Sensors and Measurements/Sequence Analyzer
  To Workspace : ToWorkspace  VariableName=Vmag4  SaveFormat=Timeseries  SampleTime=0.1
      settings: Decimation=3
  To Workspace1 : ToWorkspace  VariableName=Vmag7  SaveFormat=Timeseries  SampleTime=0.1
      settings: Decimation=3
  To Workspace10 : ToWorkspace  VariableName=Iang7  SaveFormat=Timeseries  SampleTime=0.1
      settings: Decimation=3
  To Workspace11 : ToWorkspace  VariableName=Iang9  SaveFormat=Timeseries  SampleTime=0.1
      settings: Decimation=3
  To Workspace2 : ToWorkspace  VariableName=Vmag9  SaveFormat=Timeseries  SampleTime=0.1
      settings: Decimation=3
  To Workspace3 : ToWorkspace  VariableName=Imag4  SaveFormat=Timeseries  SampleTime=0.1
      settings: Decimation=3
  To Workspace4 : ToWorkspace  VariableName=Imag7  SaveFormat=Timeseries  SampleTime=0.1
      settings: Decimation=3
  To Workspace5 : ToWorkspace  VariableName=Imag9  SaveFormat=Timeseries  SampleTime=0.1
      settings: Decimation=3
  To Workspace6 : ToWorkspace  VariableName=Vang4  SaveFormat=Timeseries  SampleTime=0.1
      settings: Decimation=3
  To Workspace7 : ToWorkspace  VariableName=Vang7  SaveFormat=Timeseries  SampleTime=0.1
      settings: Decimation=3
  To Workspace8 : ToWorkspace  VariableName=Vang9  SaveFormat=Timeseries  SampleTime=0.1
      settings: Decimation=3
  To Workspace9 : ToWorkspace  VariableName=Iang4  SaveFormat=Timeseries  SampleTime=0.1
      settings: Decimation=3
  Zero-Sequence Current : spsSequenceAnalyzerLib/Sequence Analyzer  Freq=50  n=1  seq=Zero  InInit=[1, 0]  Ts=0
      settings: LibrarySourceBlock=sps_lib/Sensors and Measurements/Sequence Analyzer
  Zero-Sequence Current 2 : spsSequenceAnalyzerLib/Sequence Analyzer  Freq=50  n=1  seq=Zero  InInit=[1, 0]  Ts=0
      settings: LibrarySourceBlock=sps_lib/Sensors and Measurements/Sequence Analyzer
  Zero-Sequence Current 3 : spsSequenceAnalyzerLib/Sequence Analyzer  Freq=50  n=1  seq=Zero  InInit=[1, 0]  Ts=0
      settings: LibrarySourceBlock=sps_lib/Sensors and Measurements/Sequence Analyzer
  Zero-Sequence Current2 : spsSequenceAnalyzerLib/Sequence Analyzer  Freq=50  n=1  seq=Zero  InInit=[1, 0]  Ts=0
      settings: LibrarySourceBlock=sps_lib/Sensors and Measurements/Sequence Analyzer
  wires:
  Positive-Sequence Current 3/3 -> Display2/1
  [Vabc_71] -> Display19/1
  [Iabc_71] -> Zero-Sequence Current 2/1, Positive-Sequence Current 2/1
  Positive-Sequence Current 3/2 -> To Workspace11/1, Display1/1
  [Vabc_81] -> Display21/1
  Positive-Sequence Current/1 -> To Workspace3/1, Scope/2, Display3/1
  Positive-Sequence Current 2/2 -> To Workspace10/1, Display7/1
  Positive-Sequence Current/2 -> To Workspace9/1, Display4/1
  [Vabc_42] -> Display14/1
  [Vabc_51] -> Display15/1
  [Iabc_41] -> Zero-Sequence Current/1, Positive-Sequence Current/1
  [Vabc_91] -> Display23/1
  Zero-Sequence Current 2/2 -> Display25/1
  Positive-Sequence Current 2/3 -> Display8/1
  [Iabc_91] -> Zero-Sequence Current 3/1, Positive-Sequence Current 3/1
  [Vabc_61] -> Display17/1
  Zero-Sequence Current/1 -> Scope/1, Display9/1
  [Vabc_41] -> Display13/1
  [Vabc_72] -> Display20/1
  [Vabc_92] -> Display24/1
  [Vabc_52] -> Display16/1
  Positive-Sequence Current/3 -> Display5/1
  [Vabc_82] -> Display22/1
  [Vabc_61] -> Display18/1
  Zero-Sequence Current/2 -> Display12/1
  Zero-Sequence Current 3/2 -> Display26/1
  Positive-Sequence Current 2/1 -> To Workspace4/1, Scope1/2, Display6/1
  Zero-Sequence Current 2/1 -> Scope1/1, Display10/1
  Positive-Sequence Current 3/1 -> To Workspace5/1, Scope2/2, Display/1
  Zero-Sequence Current 3/1 -> Scope2/1, Display11/1
  [Iabc_91] -> Display52/1
  [Iabc_82] -> Display51/1
  [Iabc_41] -> Display43/1
  [Iabc_51] -> Display44/1
  [Iabc_61] -> Display46/1
  [Iabc_81] -> Display50/1
  [Iabc_52] -> Display45/1
  [Iabc_62] -> Display47/1
  [Iabc_71] -> Display49/1
  [Iabc_71] -> Display48/1
  [Iabc_92] -> Display53/1
  [Iabc_41] -> Display42/1
  Zero-Sequence Current2/2 -> Display58/1
  Sequence Analyzer6/1 -> Scope8/1, Display57/1
  "PMU (PLL-Based, Positive-Sequence)6"/3 -> Display82/1
  Positive-Sequence Current2/3 -> Display79/1
  Sequence Analyzer6/2 -> Display61/1
  Sequence Analyzer5/1 -> Scope7/1, Display56/1
  [Vabc_91] -> Sequence Analyzer6/1, "PMU (PLL-Based, Positive-Sequence)4"/1
  "PMU (PLL-Based, Positive-Sequence)4"/3 -> Display59/1
  "PMU (PLL-Based, Positive-Sequence)6"/1 -> To Workspace1/1, Scope7/2, Display80/1
  Positive-Sequence Current2/2 -> To Workspace6/1, Display76/1
  Sequence Analyzer5/2 -> Display60/1
  Zero-Sequence Current2/1 -> Scope6/1, Display83/1
  "PMU (PLL-Based, Positive-Sequence)4"/1 -> To Workspace2/1, Scope8/2, Display54/1
  [Vabc_41] -> Zero-Sequence Current2/1, Positive-Sequence Current2/1
  "PMU (PLL-Based, Positive-Sequence)6"/2 -> To Workspace7/1, Display81/1
  "PMU (PLL-Based, Positive-Sequence)4"/2 -> To Workspace8/1, Display55/1
  [Vabc_71] -> Sequence Analyzer5/1, "PMU (PLL-Based, Positive-Sequence)6"/1
  Positive-Sequence Current2/1 -> To Workspace/1, Scope6/2, Display65/1
